simulink library "serialManipulator_lib"  (Simulink 6.3)
values from neighbouring files (symbols this model uses):
  N = size(DHpar,1)    [forwardDynamicModel.m]    (also in forwardKinematics.m; inverseDynamicModel.m; kinJacobian.m = size(DHparam,1))
  s = [s(1:end-1),s_T(i) + v_T(i)*time_int + 1/2*a_T(i)*time_int.^2 + 1/6*jerk(i)*time_int.^3]    [BAVS_genTrajectories.m]    (also in PVA.m = abs(s))
undefined symbols (not defined in the file or in its folder): Links
libraries: mblibv1 x14, simulink x3
settings Model: LastModifiedBy=MartinSvejda

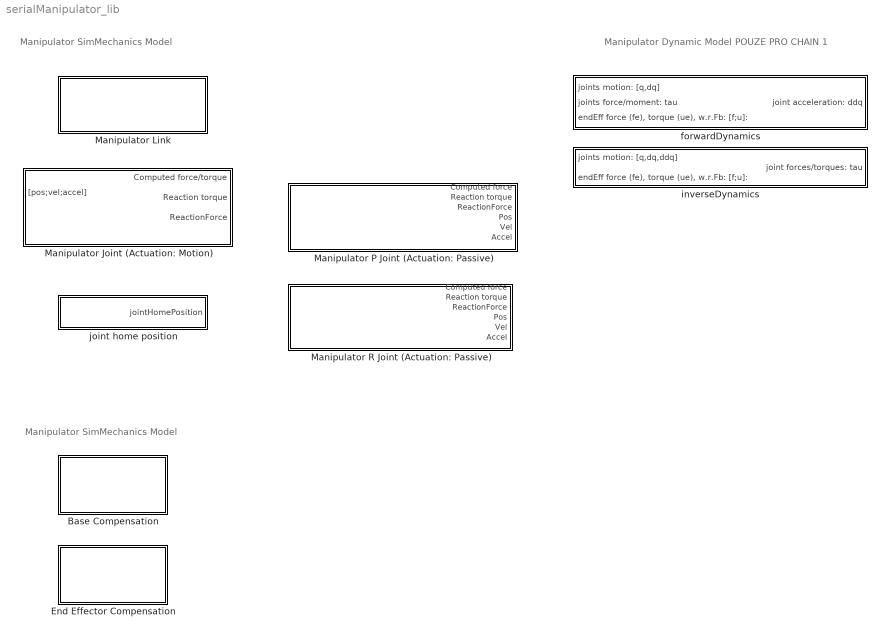
== system serialManipulator_lib ==
  note: Manipulator SimMechanics Model
  note: Manipulator Dynamic Model
      | POUZE PRO CHAIN 1
  note: Manipulator SimMechanics Model
  Base Compensation : Subsystem  mask(Links){j=1}
      mask prompts: j "Chain order"
      mask help: Base Compensation od j-th Chain
      mask Help: Kompenzace zakladny j-th Chain dane parametry Links{j}{1}
      mask Display: fprintf([num2str(j),'. Chain'])
  End Effector Compensation : Subsystem  mask(Links){j=1}
      mask prompts: j "Chain order"
      mask help: End Effector Compensation of j-th Chain
      mask Help: Kompenzace konc. ef j-th Chain dane parametry Links{j}{end}
      mask Display: fprintf([num2str(j),'. Chain'])
  Manipulator Joint (Actuation: Motion) : Subsystem  mask(Joints){j=1, i=3}
      mask prompts: j "Chain order"; i "Joint order"
      mask help: i-th ManipulatorJoint of j-th Chain
      mask Help: Vytvori R ci P kloub s prislusnym smerem osy rotace/translace z parametru ve strukture Links{j}{i}
      mask Display: fprintf(['\n',num2str(j),'. Chain \n',num2str(i),'. Joint\n'])
  Manipulator Link : Subsystem  mask(Links){j=1, i=3}
      mask prompts: j "Chain order"; i "Link order"
      mask help: i-th Manipulator Link of j-th Chain
      mask Help: Vytvori Link s prislusnymy parametry (pocatecni,koncovy bod, s.s., hmotnost, moment setrvacnosti, teziste) z parametru ve strukture Links{j}{i}
      mask Display: fprintf(['\n',num2str(j),'. Chain \n',num2str(i),'. Link\n'])
  Manipulator P Joint (Actuation: Passive) : Subsystem  mask(Joints){j=1, i=1}
      mask prompts: j "Chain order"; i "Joint order"
      mask help: PASSIVE P i-th Manipulator Joint of j-Chain
      mask Help:
      | Vytvori P kloub s prislusnym smerem osy translace z parametru ve strukture Links{j}{i} - kloub je uvazovana jako pasivni
      | 
      | Pozor, P - joint - nutno dodrzet (nekontroluje se s nastavenim v Links{j}{i) !!!
      | Nelze v SimMech vytvorit univerzalne!
      mask Display: fprintf(['\n',num2str(j),'. Chain \n',num2str(i),'. Joint\n'])
  Manipulator R Joint (Actuation: Passive) : Subsystem  AncestorBlock=|  mask(Joints){j=1, i=1}
      | serialManipulator_lib/Manipulator P Joint
      | (Actuation: Passive)
      mask prompts: j "Chain order"; i "Joint order"
      mask help: PASSIVE R i-th Manipulator Joint of j-th Chain
      mask Help:
      | Vytvori R kloub s prislusnym smerem osy rotace z parametru ve strukture Links{j}{i} - kloub je uvazovana jako pasivni
      | 
      | Pozor, R - joint - nutno dodrzet (nekontroluje se s nastavenim v Links{j}{i) !!!
      | Nelze v SimMech vytvorit univerzalne!
      mask Display: fprintf(['\n',num2str(j),'. Chain \n',num2str(i),'. Joint\n'])
  forwardDynamics : Subsystem
      mask Type: Serial Manipulator Inverse Dynamic Model
      mask Description: Inverse Dynamic Model for generalized serial manipulator
  inverseDynamics : Subsystem
      mask Type: Serial Manipulator Inverse Dynamic Model
      mask Description: Inverse Dynamic Model for generalized serial manipulator
  joint home position : Subsystem  mask(Link){j=1, i=3}
      mask prompts: j "Chain order"; i "Joint order"
      mask help: i-th joint home position
      mask Display: fprintf(['\n',num2str(j),'. Chain \n',num2str(i),'. Link\n'])

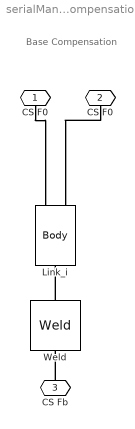
== system serialManipulator_lib/Base Compensation ==
  note: Base Compensation
  Link_i : mblibv1/Bodies/Body  Orientation=up  PhysicalDomain=mechanical  SubClassName=Unknown  LeftPortType=workingframe  RightPortType=workingframe  LConnTagsString=CS1  RConnTagsString=CS2|CS3  DialogClass=MechanicalBodyBlock  Mass=1e-10  MassUnits=kg  InertiaUnits=kg*m^2  Inertia=1e-10*eye(3)  Shape=Cylinder  ShapeDims=[1 1]  ShapeUnits=m  ShapeUse=false  Density=1  DensityUnits=kg/m^3  DensityUse=false  CG=Left$CG$Links{j}{1}.A$WORLD$WORLD$m$Links{j}{1}.R$3x3 Transform$deg$WORLD$false  WorkingFrames=Left$CS1$Links{j}{1}.A$WORLD$WORLD$m$Links{j}{1}.R$3x3 Transform$deg$WORLD$true#Right$CS2$Links{j}{1}.B$WORLD$WORLD$m$Links{j}{1}.R$3x3 Transform$deg$WORLD$true#Right$CS3$Links{j}{1}.B$WORLD$WORLD$m$Links{j}{1}.R$3x3 Transform$deg$WORLD$true
  Weld : mblibv1/Joints/Weld  Orientation=up  PhysicalDomain=mechanical  SubClassName=Unknown  LeftPortType=blob  RightPortType=blob  LConnTagsString=__newl0  RConnTagsString=__newr0  NumSAPorts=0  CutJoint=off  MarkAsCut=off  Primitives=weld  PrimitiveProps=W$INERTIAL$[0 0 0]$weld  DialogClass=JointBlock
  CS F0 : PMIOPort  Orientation=down  Port=1  Side=Right
  " CS F0" : PMIOPort  Orientation=down  Port=2  Side=Right
  CS Fb : PMIOPort  Orientation=up  Port=3  Side=Left
  connections:
  " CS F0"/RConn1 -- Link_i/RConn2
  CS F0/RConn1 -- Link_i/RConn1
  CS Fb/RConn1 -- Weld/LConn1
  Weld/RConn1 -- Link_i/LConn1

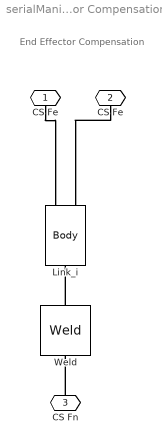
== system serialManipulator_lib/End Effector Compensation ==
  note: End Effector Compensation
  Link_i : mblibv1/Bodies/Body  Orientation=up  PhysicalDomain=mechanical  SubClassName=Unknown  LeftPortType=workingframe  RightPortType=workingframe  LConnTagsString=CS1  RConnTagsString=CS2|CS3  DialogClass=MechanicalBodyBlock  Mass=1e-10  MassUnits=kg  InertiaUnits=kg*m^2  Inertia=1e-10*eye(3)  Shape=Cylinder  ShapeDims=[1 1]  ShapeUnits=m  ShapeUse=false  Density=1  DensityUnits=kg/m^3  DensityUse=false  CG=Left$CG$Links{j}{end}.A$WORLD$WORLD$m$Links{j}{end}.R$3x3 Transform$deg$WORLD$false  WorkingFrames=Left$CS1$Links{j}{end}.A$WORLD$WORLD$m$Links{j}{end}.R$3x3 Transform$deg$WORLD$true#Right$CS2$Links{j}{end}.B$WORLD$WORLD$m$Links{j}{end}.R$3x3 Transform$deg$WORLD$true#Right$CS3$Links{j}{end}.B$WORLD$WORLD$m$Links{j}{end}.R$3x3 Transform$deg$WORLD$true
  Weld : mblibv1/Joints/Weld  Orientation=up  PhysicalDomain=mechanical  SubClassName=Unknown  LeftPortType=blob  RightPortType=blob  LConnTagsString=__newl0  RConnTagsString=__newr0  NumSAPorts=0  CutJoint=off  MarkAsCut=off  Primitives=weld  PrimitiveProps=W$INERTIAL$[0 0 0]$weld  DialogClass=JointBlock
  CS Fe : PMIOPort  Orientation=down  Port=1  Side=Right
  " CS Fe" : PMIOPort  Orientation=down  Port=2  Side=Right
  CS Fn : PMIOPort  Orientation=up  Port=3  Side=Left
  connections:
  " CS Fe"/RConn1 -- Link_i/RConn2
  CS Fe/RConn1 -- Link_i/RConn1
  CS Fn/RConn1 -- Weld/LConn1
  Weld/RConn1 -- Link_i/LConn1

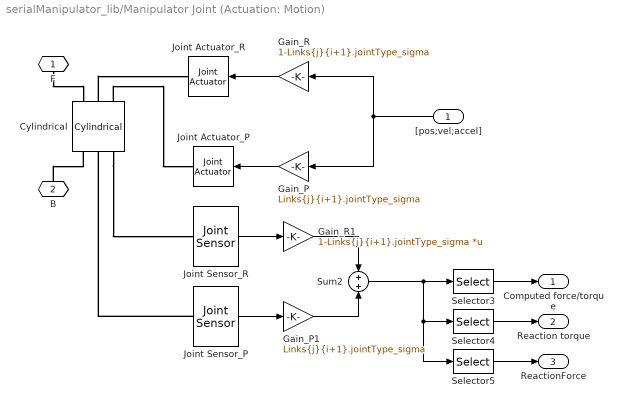
== system serialManipulator_lib/Manipulator Joint (Actuation: Motion) ==
  "[pos;vel;accel]" : Inport  Orientation=left
  Cylindrical : mblibv1/Joints/Cylindrical  Orientation=up  PhysicalDomain=mechanical  SubClassName=Unknown  LeftPortType=blob  RightPortType=blob  LConnTagsString=__newl0|SA1|SA2  RConnTagsString=__newr0|SA1|SA2  NumSAPorts=4  CutJoint=off  MarkAsCut=off  Primitives=prismatic_revolute  PrimitiveProps=P1$WORLD$Links{j}{i+1}.jointAxis$prismatic#R1$WORLD$Links{j}{i+1}.jointAxis$revolute  DialogClass=JointBlock
  Gain_P : Gain  Orientation=left  Gain=Links{j}{i+1}.jointType_sigma
  Gain_P1 : Gain  Gain=Links{j}{i+1}.jointType_sigma
  Gain_R : Gain  Orientation=left  Gain=1-Links{j}{i+1}.jointType_sigma
  Gain_R1 : Gain  Gain=1-Links{j}{i+1}.jointType_sigma  Multiplication=Matrix(K*u)
  Joint Actuator_P : mblibv1/Sensors &  Actuators/Joint Actuator  Orientation=left  PhysicalDomain=Mechanical  PortType=blob  ActuationStyle=Motion  AngleUnits=rad  ArcVelocityUnits=rad/s  ArcAccelerationUnits=rad/s^2  CoordPositionUnits=m  VelocityUnits=m/s  AccelerationUnits=m/s^2  ForceUnits=N  TorqueUnits=N-m  ActiveIO=off  Width=3  DialogClass=MechanicalActuatorBlock  Primitive=P1  ReferenceFrame=Absolute (INERTIAL)
  Joint Actuator_R : mblibv1/Sensors &  Actuators/Joint Actuator  Orientation=left  PhysicalDomain=Mechanical  PortType=blob  ActuationStyle=Motion  AngleUnits=rad  ArcVelocityUnits=rad/s  ArcAccelerationUnits=rad/s^2  CoordPositionUnits=m  VelocityUnits=m/s  AccelerationUnits=m/s^2  ForceUnits=N  TorqueUnits=N-m  ActiveIO=off  Width=3  DialogClass=MechanicalActuatorBlock  Primitive=R1  ReferenceFrame=Absolute (INERTIAL)
  Joint Sensor_P : mblibv1/Sensors &  Actuators/Joint Sensor  PhysicalDomain=Mechanical  PortType=blob  Muxed=on  Pose=off  Angle=off  AngleUnits=rad  ArcVelocity=off  ArcVelocityUnits=rad/s  ArcAcceleration=off  ArcAccelerationUnits=rad/s^2  CoordPosition=off  CoordPositionUnits=m  Velocity=off  VelocityUnits=m/s  Acceleration=off  AccelerationUnits=m/s^2  Quaternion=on  QuaternionDT=off  QuaternionDDT=off  QuaternionUnits=off  OutputVector=[ 1 3 3 ]  ActiveIO=off  Width=7  DialogClass=MechanicalSensorBlock  Primitive=P1  Force=on  ForceUnits=N  Torque=on  TorqueUnits=N-m  ReferenceFrame=Absolute (INERTIAL)  ReactionSensedSide=Base  ReactionReferenceFrame=Absolute (World)  ReactionForce=on  ReactionForceUnits=N  ReactionMoment=on  ReactionMomentUnits=N-m
  Joint Sensor_R : mblibv1/Sensors &  Actuators/Joint Sensor  PhysicalDomain=Mechanical  PortType=blob  Muxed=on  Pose=off  Angle=off  AngleUnits=rad  ArcVelocity=off  ArcVelocityUnits=rad/s  ArcAcceleration=off  ArcAccelerationUnits=rad/s^2  CoordPosition=off  CoordPositionUnits=m  Velocity=off  VelocityUnits=m/s  Acceleration=off  AccelerationUnits=m/s^2  Quaternion=on  QuaternionDT=off  QuaternionDDT=off  QuaternionUnits=off  OutputVector=[ 1 3 3 ]  ActiveIO=off  Width=7  DialogClass=MechanicalSensorBlock  Primitive=R1  Force=on  ForceUnits=N  Torque=on  TorqueUnits=N-m  ReferenceFrame=Absolute (INERTIAL)  ReactionSensedSide=Base  ReactionReferenceFrame=Absolute (World)  ReactionForce=on  ReactionForceUnits=N  ReactionMoment=on  ReactionMomentUnits=N-m
  Selector3 : Selector  Elements=[1]  Columns=7  InputPortWidth=7
  Selector4 : Selector  Elements=[2:4]  Columns=7  InputPortWidth=7
  Selector5 : Selector  Elements=[5:7]  Columns=7  InputPortWidth=7
  Sum2 : Sum
  F : PMIOPort  Orientation=down  Port=1  Side=Right
  B : PMIOPort  Orientation=up  Port=2  Side=Left
  Computed force/torque : Outport
  Reaction torque : Outport  Port=2
  ReactionForce : Outport  Port=3
  wires:
  Gain_R/1 -> Joint Actuator_R/1
  Gain_P/1 -> Joint Actuator_P/1
  Joint Sensor_R/1 -> Gain_R1/1
  Gain_P1/1 -> Sum2/2
  Gain_R1/1 -> Sum2/1
  Joint Sensor_P/1 -> Gain_P1/1
  Sum2/1 -> Selector3/1, Selector4/1, Selector5/1
  Selector3/1 -> Computed force/torque/1
  Selector4/1 -> Reaction torque/1
  Selector5/1 -> ReactionForce/1
  "[pos;vel;accel]"/1 -> Gain_P/1, Gain_R/1
  connections:
  Joint Sensor_P/LConn1 -- Cylindrical/LConn2
  Cylindrical/LConn3 -- Joint Sensor_R/LConn1
  Cylindrical/RConn2 -- Joint Actuator_R/RConn1
  Cylindrical/RConn3 -- Joint Actuator_P/RConn1
  F/RConn1 -- Cylindrical/RConn1
  B/RConn1 -- Cylindrical/LConn1

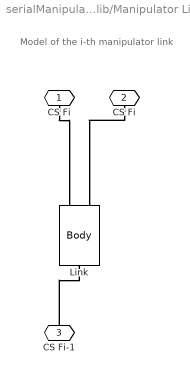
== system serialManipulator_lib/Manipulator Link ==
  note: Model of the i-th manipulator link
  Link : mblibv1/Bodies/Body  Orientation=up  PhysicalDomain=mechanical  SubClassName=Unknown  LeftPortType=workingframe  RightPortType=workingframe  LConnTagsString=CS1  RConnTagsString=CS2|CS3  DialogClass=MechanicalBodyBlock  Mass=Links{j}{i+1}.mass  MassUnits=kg  InertiaUnits=kg*m^2  Inertia=Links{j}{i+1}.inertiaTensor  Shape=Cylinder  ShapeDims=[1 1]  ShapeUnits=m  ShapeUse=false  Density=1  DensityUnits=kg/m^3  DensityUse=false  CG=Left$CG$Links{j}{i+1}.gravityCenter$WORLD$WORLD$m$Links{j}{i+1}.R$3x3 Transform$deg$WORLD$false  WorkingFrames=Left$CS1$Links{j}{i+1}.A$WORLD$WORLD$m$Links{j}{i+1}.R$3x3 Transform$deg$WORLD$true#Right$CS2$Links{j}{i+1}.B$WORLD$WORLD$m$Links{j}{i+1}.R$3x3 Transform$deg$WORLD$true#Right$CS3$Links{j}{i+1}.B$WORLD$WORLD$m$Links{j}{i+1}.R$3x3 Transform$deg$WORLD$true
  CS Fi : PMIOPort  Orientation=down  Port=1  Side=Right
  " CS Fi" : PMIOPort  Orientation=down  Port=2  Side=Right
  CS Fi-1 : PMIOPort  Orientation=up  Port=3  Side=Left
  connections:
  CS Fi/RConn1 -- Link/RConn1
  " CS Fi"/RConn1 -- Link/RConn2
  CS Fi-1/RConn1 -- Link/LConn1

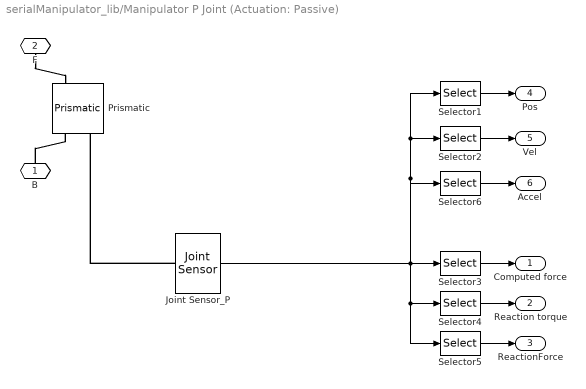
== system serialManipulator_lib/Manipulator P Joint (Actuation: Passive) ==
  Joint Sensor_P : mblibv1/Sensors &  Actuators/Joint Sensor  PhysicalDomain=Mechanical  PortType=blob  Muxed=on  Pose=off  Angle=off  AngleUnits=rad  ArcVelocity=off  ArcVelocityUnits=rad/s  ArcAcceleration=off  ArcAccelerationUnits=rad/s^2  CoordPosition=on  CoordPositionUnits=m  Velocity=on  VelocityUnits=m/s  Acceleration=on  AccelerationUnits=m/s^2  Quaternion=on  QuaternionDT=off  QuaternionDDT=off  OutputVector=[ 1 1 1 1 3 3 ]  ActiveIO=off  Width=7  DialogClass=MechanicalSensorBlock  Primitive=P1  Force=on  ForceUnits=N  Torque=on  TorqueUnits=N-m  ReferenceFrame=Absolute (INERTIAL)  ReactionSensedSide=Base  ReactionReferenceFrame=Absolute (World)  ReactionForce=on  ReactionForceUnits=N  ReactionMoment=on  ReactionMomentUnits=N-m
  Prismatic : mblibv1/Joints/Prismatic  Orientation=up  PhysicalDomain=mechanical  SubClassName=Unknown  LeftPortType=blob  RightPortType=blob  LConnTagsString=__newl0|SA1  RConnTagsString=__newr0|SA1  NumSAPorts=2  CutJoint=off  MarkAsCut=off  Primitives=prismatic  PrimitiveProps=P1$WORLD$Links{j}{i+1}.jointAxis$prismatic  DialogClass=JointBlock
  Selector1 : Selector  Elements=[1]  Columns=7  InputPortWidth=10
  Selector2 : Selector  Elements=[2]  Columns=7  InputPortWidth=10
  Selector3 : Selector  Elements=[4]  Columns=7  InputPortWidth=10
  Selector4 : Selector  Elements=[5:7]  Columns=7  InputPortWidth=10
  Selector5 : Selector  Elements=[8:10]  Columns=7  InputPortWidth=10
  Selector6 : Selector  Elements=[3]  Columns=7  InputPortWidth=10
  B : PMIOPort  Orientation=up  Port=1  Side=Left
  F : PMIOPort  Orientation=down  Port=2  Side=Right
  Computed force : Outport
  Reaction torque : Outport  Port=2
  ReactionForce : Outport  Port=3
  Pos : Outport  Port=4
  Vel : Outport  Port=5
  Accel : Outport  Port=6
  wires:
  Selector3/1 -> Computed force/1
  Selector4/1 -> Reaction torque/1
  Selector5/1 -> ReactionForce/1
  Joint Sensor_P/1 -> Selector3/1, Selector4/1, Selector5/1, Selector1/1, Selector2/1, Selector6/1
  Selector1/1 -> Pos/1
  Selector2/1 -> Vel/1
  Selector6/1 -> Accel/1
  connections:
  B/RConn1 -- Prismatic/LConn1
  F/RConn1 -- Prismatic/RConn1
  Joint Sensor_P/LConn1 -- Prismatic/LConn2

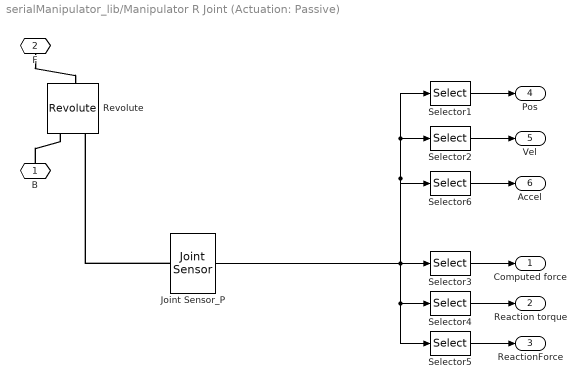
== system serialManipulator_lib/Manipulator R Joint (Actuation: Passive) ==
  Joint Sensor_P : mblibv1/Sensors &  Actuators/Joint Sensor  PhysicalDomain=Mechanical  PortType=blob  Muxed=on  Pose=off  Angle=on  AngleUnits=rad  ArcVelocity=on  ArcVelocityUnits=rad/s  ArcAcceleration=on  ArcAccelerationUnits=rad/s^2  CoordPosition=on  CoordPositionUnits=m  Velocity=off  VelocityUnits=m/s  Acceleration=off  AccelerationUnits=m/s^2  Quaternion=on  QuaternionDT=off  QuaternionDDT=off  OutputVector=[ 1 1 1 1 3 3 ]  ActiveIO=off  Width=7  DialogClass=MechanicalSensorBlock  Primitive=R1  Force=on  ForceUnits=N  Torque=on  TorqueUnits=N-m  ReferenceFrame=Absolute (INERTIAL)  ReactionSensedSide=Base  ReactionReferenceFrame=Absolute (World)  ReactionForce=on  ReactionForceUnits=N  ReactionMoment=on  ReactionMomentUnits=N-m
  Revolute : mblibv1/Joints/Revolute  Orientation=up  PhysicalDomain=mechanical  SubClassName=Unknown  LeftPortType=blob  RightPortType=blob  LConnTagsString=__newl0|SA1  RConnTagsString=__newr0  NumSAPorts=1  CutJoint=off  MarkAsCut=off  Primitives=revolute  PrimitiveProps=R1$WORLD$Links{j}{i+1}.jointAxis$revolute  DialogClass=JointBlock
  Selector1 : Selector  Elements=[1]  Columns=7  InputPortWidth=10
  Selector2 : Selector  Elements=[2]  Columns=7  InputPortWidth=10
  Selector3 : Selector  Elements=[4]  Columns=7  InputPortWidth=10
  Selector4 : Selector  Elements=[5:7]  Columns=7  InputPortWidth=10
  Selector5 : Selector  Elements=[8:10]  Columns=7  InputPortWidth=10
  Selector6 : Selector  Elements=[3]  Columns=7  InputPortWidth=10
  B : PMIOPort  Orientation=up  Port=1  Side=Left
  F : PMIOPort  Orientation=down  Port=2  Side=Right
  Computed force : Outport
  Reaction torque : Outport  Port=2
  ReactionForce : Outport  Port=3
  Pos : Outport  Port=4
  Vel : Outport  Port=5
  Accel : Outport  Port=6
  wires:
  Selector3/1 -> Computed force/1
  Selector4/1 -> Reaction torque/1
  Selector5/1 -> ReactionForce/1
  Joint Sensor_P/1 -> Selector3/1, Selector4/1, Selector5/1, Selector1/1, Selector2/1, Selector6/1
  Selector1/1 -> Pos/1
  Selector2/1 -> Vel/1
  Selector6/1 -> Accel/1
  connections:
  Joint Sensor_P/LConn1 -- Revolute/LConn2
  F/RConn1 -- Revolute/RConn1
  B/RConn1 -- Revolute/LConn1

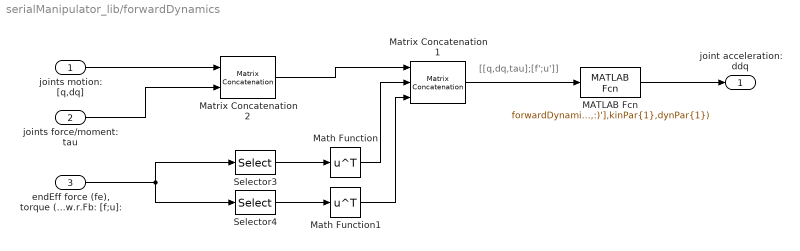
== system serialManipulator_lib/forwardDynamics ==
  note: [[q,dq,tau];[f';u']]
  joints motion: [q,dq] : Inport
  joints force/moment: tau : Inport  Port=2
  "endEff force (fe), torque (ue), w.r.Fb: [f;u]:" : Inport  Port=3
  MATLAB Fcn : MATLABFcn  MATLABFcn=forwardDynamicModel(u(1:end-2,1:2),u(1:end-2,3),[u(end-1,:)';u(end,:)'],kinPar{1},dynPar{1})  OutputDimensions=[Links{1}{1}.numOfLinks]  Output1D=off
  Math Function : Math  Operator=transpose  SaturateOnIntegerOverflow=on
  Math Function1 : Math  Operator=transpose  SaturateOnIntegerOverflow=on
  Matrix Concatenation1 : simulink/Math Operations/Matrix Concatenation  numInports=3  catMethod=Vertical
  Matrix Concatenation2 : simulink/Math Operations/Matrix Concatenation  numInports=2  catMethod=Horizontal
  Selector3 : Selector  InputType=Matrix  Elements=[:,1]  Rows=1:3  InputPortWidth=6
  Selector4 : Selector  InputType=Matrix  Elements=[:,1]  Rows=4:6  InputPortWidth=6
  joint acceleration: ddq : Outport
  wires:
  joints force/moment: tau/1 -> Matrix Concatenation2/2
  Matrix Concatenation2/1 -> Matrix Concatenation1/1
  joints motion: [q,dq]/1 -> Matrix Concatenation2/1
  Math Function/1 -> Matrix Concatenation1/2
  Selector3/1 -> Math Function/1
  Selector4/1 -> Math Function1/1
  Math Function1/1 -> Matrix Concatenation1/3
  Matrix Concatenation1/1 -> MATLAB Fcn/1
  "endEff force (fe), torque (ue), w.r.Fb: [f;u]:"/1 -> Selector4/1, Selector3/1
  MATLAB Fcn/1 -> joint acceleration: ddq/1

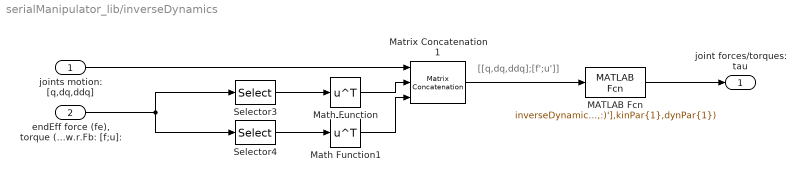
== system serialManipulator_lib/inverseDynamics ==
  note: [[q,dq,ddq];[f';u']]
  joints motion: [q,dq,ddq] : Inport
  "endEff force (fe), torque (ue), w.r.Fb: [f;u]:" : Inport  Port=2
  MATLAB Fcn : MATLABFcn  MATLABFcn=inverseDynamicModel(u(1:end-2,:),[u(end-1,:)';u(end,:)'],kinPar{1},dynPar{1})  Output1D=off
  Math Function : Math  Operator=transpose  SaturateOnIntegerOverflow=on
  Math Function1 : Math  Operator=transpose  SaturateOnIntegerOverflow=on
  Matrix Concatenation1 : simulink/Math Operations/Matrix Concatenation  numInports=3  catMethod=Vertical
  Selector3 : Selector  InputType=Matrix  Elements=[:,1]  Rows=1:3  InputPortWidth=6
  Selector4 : Selector  InputType=Matrix  Elements=[:,1]  Rows=4:6  InputPortWidth=6
  joint forces/torques: tau : Outport
  wires:
  Math Function/1 -> Matrix Concatenation1/2
  Selector3/1 -> Math Function/1
  Selector4/1 -> Math Function1/1
  Math Function1/1 -> Matrix Concatenation1/3
  Matrix Concatenation1/1 -> MATLAB Fcn/1
  "endEff force (fe), torque (ue), w.r.Fb: [f;u]:"/1 -> Selector4/1, Selector3/1
  joints motion: [q,dq,ddq]/1 -> Matrix Concatenation1/1
  MATLAB Fcn/1 -> joint forces/torques: tau/1

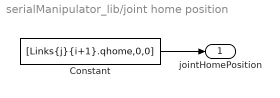
== system serialManipulator_lib/joint home position ==
  Constant : Constant  Value=[Links{j}{i+1}.qhome,0,0]
  jointHomePosition : Outport
  wires:
  Constant/1 -> jointHomePosition/1
